simulink model "VehDyn_nstm_model"  (R2023a)
settings: Solver=ode4  StartTime=0.0  StopTime=tend  FixedStep=sample_Ti  RelTol=1e-3
values from neighbouring files (symbols this model uses):
  dpsi_rad_INIT = data.dpsi_radps(1)    [load_nstm_withSimData.m]
  omega_rad_INIT = data.vx_mps(1)/tireFL__MFSIMPLE__r_tire_m    [load_nstm_withSimData.m]
  sample_Ti = 1.e-3    (= 0.001)    [load_nstm_withSimData.m]
  tireFL__MFSIMPLE__r_tire_m = 0.3118    [VehParams.m]
  tireRL__MFSIMPLE__r_tire_m = 0.3118    [VehParams.m]
  VEH__Brakes__d_BrakeActuatorBoreFrRe_m__1 = 0.0798    [VehParams.m]
  VEH__Brakes__d_BrakeActuatorBoreFrRe_m__2 = 0.0798    [VehParams.m]
  VEH__Brakes__mue_BrakePadsFrRe_kinetic__1 = 0.4    [VehParams.m]
  VEH__Brakes__mue_BrakePadsFrRe_kinetic__2 = 0.4    [VehParams.m]
  VEH__Brakes__n_BrakePadsNumberFrRe__1 = 1    [VehParams.m]
  VEH__Brakes__n_BrakePadsNumberFrRe__2 = 1    [VehParams.m]
  VEH__Brakes__r_BrakePadsMeanLeverFrRe_m__1 = 0.134    [VehParams.m]
  VEH__Brakes__r_BrakePadsMeanLeverFrRe_m__2 = 0.134    [VehParams.m]
  VEH__STMspecific__switchModelVel_mps = 3    [VehParams.m]
  vx_INIT = data.vx_mps(1)    [load_nstm_withSimData.m]
  vy_INIT = data.vy_mps(1)    [load_nstm_withSimData.m]
  x0_positionstates = [0 0 0]    [VehParams.m]
  x0_stm_vehiclestates = [0; 0; 0; 0; 0; 0; 0; 0]    [VehParams.m]
settings Model: Creator=ADMIN  LastModifiedBy=ADMIN

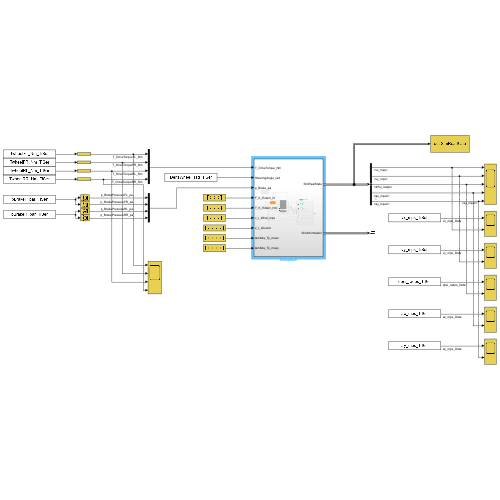
[thumbnail: Simulink's stored preview of the top-level diagram]
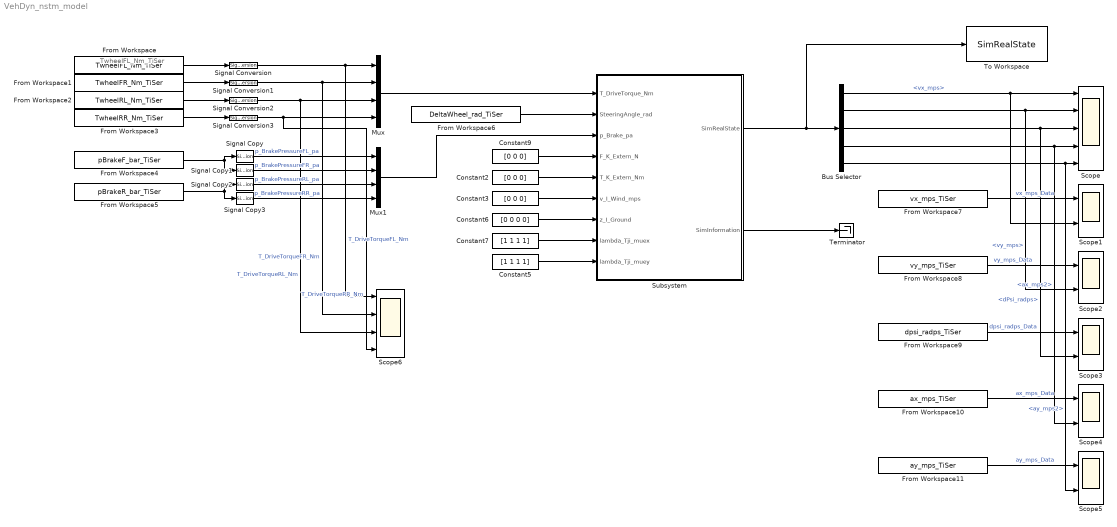
== system VehDyn_nstm_model ==
  note: TwheelFL_Nm_TiSer
  Bus Selector : BusSelector  OutputSignals=vx_mps,vy_mps,dPsi_radps,ax_mps2,ay_mps2
  Constant2 : Constant  Value=[0 0 0]
  Constant3 : Constant  Value=[0 0 0]
  Constant5 : Constant  Value=[1 1 1 1]
  Constant6 : Constant  Value=[0 0 0 0]
  Constant7 : Constant  Value=[1 1 1 1]
  Constant9 : Constant  Value=[0 0 0]
  From Workspace : FromWorkspace  VariableName=TwheelFL_Nm_TiSer  SampleTime=sample_Ti
  From Workspace1 : FromWorkspace  VariableName=TwheelFR_Nm_TiSer  SampleTime=sample_Ti
  From Workspace10 : FromWorkspace  VariableName=ax_mps_TiSer  SampleTime=sample_Ti
  From Workspace11 : FromWorkspace  VariableName=ay_mps_TiSer  SampleTime=sample_Ti
  From Workspace2 : FromWorkspace  VariableName=TwheelRL_Nm_TiSer  SampleTime=sample_Ti
  From Workspace3 : FromWorkspace  VariableName=TwheelRR_Nm_TiSer  SampleTime=sample_Ti
  From Workspace4 : FromWorkspace  VariableName=pBrakeF_bar_TiSer  SampleTime=sample_Ti
  From Workspace5 : FromWorkspace  VariableName=pBrakeR_bar_TiSer  SampleTime=sample_Ti
  From Workspace6 : FromWorkspace  VariableName=DeltaWheel_rad_TiSer  SampleTime=sample_Ti
  From Workspace7 : FromWorkspace  VariableName=vx_mps_TiSer  SampleTime=sample_Ti
  From Workspace8 : FromWorkspace  VariableName=vy_mps_TiSer  SampleTime=sample_Ti
  From Workspace9 : FromWorkspace  VariableName=dpsi_radps_TiSer  SampleTime=sample_Ti
  Mux : Mux
  Mux1 : Mux
  Scope : Scope  NumInputPorts=5
  Scope{1..5} (5 alike) : Scope  NumInputPorts=2
  Scope6 : Scope  NumInputPorts=4
  Signal Conversion{,1..3} (4 alike) : SignalConversion  OverrideOpt=off
  Signal Copy{,1..3} (4 alike) : SignalConversion  OverrideOpt=off
  Subsystem : Subsystem
  Terminator : Terminator
  To Workspace : ToWorkspace  VariableName=SimRealState  SaveFormat=Timeseries  SampleTime=sample_Ti
  wires:
  Signal Copy2/1 -> Mux1/3  "p_BrakePressureRL_pa"
  From Workspace/1 -> Signal Conversion/1
  Mux1/1 -> Subsystem/3(p_Brake_pa)
  From Workspace1/1 -> Signal Conversion1/1
  Signal Conversion/1 -> Scope6/1, Mux/1  "T_DriveTorqueFL_Nm"
  Subsystem/2(SimInformation) -> Terminator/1
  Signal Copy1/1 -> Mux1/2  "p_BrakePressureFR_pa"
  From Workspace3/1 -> Signal Conversion3/1
  From Workspace4/1 -> Signal Copy1/1, Signal Copy/1
  Signal Copy/1 -> Mux1/1  "p_BrakePressureFL_pa"
  From Workspace5/1 -> Signal Copy2/1, Signal Copy3/1
  Bus Selector/1 -> Scope1/2, Scope/1  "<vx_mps>"
  From Workspace2/1 -> Signal Conversion2/1
  Constant2/1 -> Subsystem/5(T_K_Extern_Nm)
  Constant5/1 -> Subsystem/9(lambda_Tji_muey)
  Constant9/1 -> Subsystem/4(F_K_Extern_N)
  Subsystem/1(SimRealState) -> To Workspace/1, Bus Selector/1
  Signal Copy3/1 -> Mux1/4  "p_BrakePressureRR_pa"
  Constant6/1 -> Subsystem/7(z_I_Ground)
  Constant3/1 -> Subsystem/6(v_I_Wind_mps)
  From Workspace6/1 -> Subsystem/2(SteeringAngle_rad)
  Signal Conversion3/1 -> Scope6/4, Mux/4  "T_DriveTorqueRR_Nm"
  Mux/1 -> Subsystem/1(T_DriveTorque_Nm)
  Signal Conversion2/1 -> Scope6/3, Mux/3  "T_DriveTorqueRL_Nm"
  Constant7/1 -> Subsystem/8(lambda_Tji_muex)
  Signal Conversion1/1 -> Scope6/2, Mux/2  "T_DriveTorqueFR_Nm"
  From Workspace7/1 -> Scope1/1  "vx_mps_Data"
  From Workspace8/1 -> Scope2/1  "vy_mps_Data"
  Bus Selector/2 -> Scope2/2, Scope/2  "<vy_mps>"
  From Workspace9/1 -> Scope3/1  "dpsi_radps_Data"
  Bus Selector/3 -> Scope3/2, Scope/3  "<dPsi_radps>"
  Bus Selector/4 -> Scope4/2, Scope/4  "<ax_mps2>"
  From Workspace10/1 -> Scope4/1  "ax_mps_Data"
  From Workspace11/1 -> Scope5/1  "ay_mps_Data"
  Bus Selector/5 -> Scope5/2, Scope/5  "<ay_mps2>"

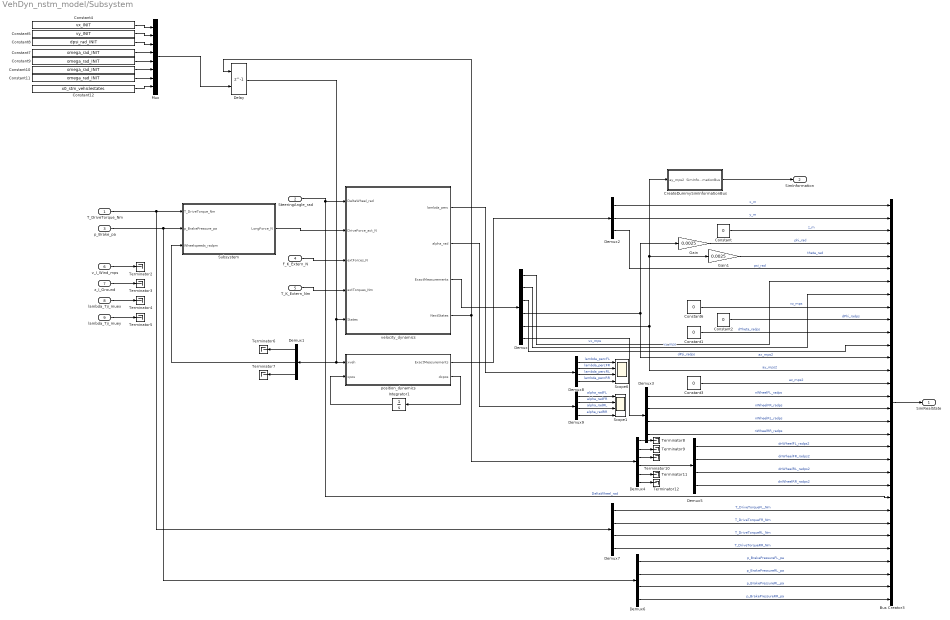
== system VehDyn_nstm_model/Subsystem ==
  T_DriveTorque_Nm : Inport
  SteeringAngle_rad : Inport  Port=2
  p_Brake_pa : Inport  Port=3
  F_K_Extern_N : Inport  Port=4  PortDimensions=3
  T_K_Extern_Nm : Inport  Port=5  PortDimensions=3
  v_I_Wind_mps : Inport  Port=6  PortDimensions=3
  z_I_Ground : Inport  Port=7  PortDimensions=4
  lambda_Tji_muex : Inport  Port=8  PortDimensions=4
  lambda_Tji_muey : Inport  Port=9  PortDimensions=4
  Bus Creator3 : BusCreator  Inputs=32  OutDataTypeStr=Bus: SimRealState
      settings: InheritFromInputs=off
  Constant{,1..3,6} (5 alike) : Constant  Value=0
  Constant{7,9..11} (4 alike) : Constant  Value=omega_rad_INIT
  Constant12 : Constant  Value=x0_stm_vehiclestates
  Constant4 : Constant  Value=vx_INIT
  Constant5 : Constant  Value=vy_INIT
  Constant8 : Constant  Value=dpsi_rad_INIT
  CreateDummySimInformationBus : Subsystem
  Delay : Delay  DelayLength=1  InitialConditionSource=Input port  InitialCondition=0
      settings: InputPortMap=u0,p4
  Demux : Demux  Outputs=[1 1 1 1 1 4]
  Demux1 : Demux  Outputs=[3 4 8]
  Demux2 : Demux  Outputs=3
  Demux{3,5..9} (6 alike) : Demux
  Demux4 : Demux  Outputs=[1 1 1 4 4 4]
  Gain : Gain  Gain=0.0025
  Gain1 : Gain  Gain=0.0025
  Integrator1 : Integrator  InitialCondition=x0_positionstates
  Mux : Mux  Inputs=8
  Scope1 : Scope  NumInputPorts=4
  Scope6 : Scope  NumInputPorts=4
  Subsystem : Subsystem
  Terminator{2..12} (11 alike) : Terminator
  position_dynamics : MATLAB Function  TreatAsAtomicUnit=on
  velocity_dynamics : MATLAB Function  TreatAsAtomicUnit=on
  SimRealState : Outport  OutDataTypeStr=Bus: SimRealState  SampleTime=sample_Ti  VectorParamsAs1DForOutWhenUnconnected=off
  SimInformation : Outport  Port=2  OutDataTypeStr=Bus: SimInformation  VectorParamsAs1DForOutWhenUnconnected=off
  wires:
  Demux2/1 -> Bus Creator3/1  "x_m"
  Demux4/2 -> Terminator9/1
  Constant12/1 -> Mux/8
  Demux/4 -> Gain/1, Bus Creator3/13  "ax_mps2"
  Subsystem/1(LongForce_N) -> velocity_dynamics/2(DriveForce_act_N)
  Bus Creator3/1 -> SimRealState/1
  F_K_Extern_N/1 -> velocity_dynamics/3(extForces_N)
  Constant1/1 -> Bus Creator3/11  "dTheta_radps"
  Demux7/1 -> Bus Creator3/25  "T_DriveTorqueFL_Nm"
  Constant10/1 -> Mux/6
  Constant6/1 -> Bus Creator3/9  "vz_mps"
  Constant8/1 -> Mux/3
  z_I_Ground/1 -> Terminator3/1
  Demux7/4 -> Bus Creator3/28  "T_DriveTorqueRR_Nm"
  Demux7/2 -> Bus Creator3/26  "T_DriveTorqueFR_Nm"
  position_dynamics/1(ExactMeasurements) -> Demux2/1
  Constant4/1 -> Mux/1
  Constant9/1 -> Mux/5
  Demux4/4 -> Demux5/1
  Demux/3 -> Bus Creator3/12  "dPsi_radps"
  Demux6/3 -> Bus Creator3/31  "p_BrakePressureRL_pa"
  CreateDummySimInformationBus/1(SimInformationBus) -> SimInformation/1
  Gain1/1 -> Bus Creator3/5  "theta_rad"
  Constant5/1 -> Mux/2
  Mux/1 -> Delay/2
  p_Brake_pa/1 -> Subsystem/2(p_BrakePressure_pa), Demux6/1
  Demux2/2 -> Bus Creator3/2  "y_m"
  velocity_dynamics/3(ExactMeasurements) -> Demux/1
  Demux5/4 -> Bus Creator3/23  "dnWheelRR_radps2"
  lambda_Tji_muey/1 -> Terminator5/1
  velocity_dynamics/4(NextStates) -> Delay/1, Demux4/1
  Demux1/1 -> Terminator6/1
  Demux4/6 -> Terminator12/1
  Demux4/5 -> Terminator11/1
  Demux4/1 -> Terminator8/1
  lambda_Tji_muex/1 -> Terminator4/1
  Demux3/4 -> Bus Creator3/19  "nWheelRR_radps"
  Demux6/1 -> Bus Creator3/29  "p_BrakePressureFL_pa"
  Demux1/2 -> Subsystem/3(Wheelspeeds_radpm)
  Demux2/3 -> Bus Creator3/6  "psi_rad"
  Demux6/4 -> Bus Creator3/32  "p_BrakePressureRR_pa"
  Constant3/1 -> Bus Creator3/15  "az_mps2"
  Demux6/2 -> Bus Creator3/30  "p_BrakePressureRL_pa"
  Demux5/1 -> Bus Creator3/20  "dnWheelFL_radps2"
  Demux5/2 -> Bus Creator3/21  "dnWheelFR_radps2"
  Demux/1 -> Bus Creator3/7  "vx_mps"
  SteeringAngle_rad/1 -> Bus Creator3/24, velocity_dynamics/1(DeltaWheel_rad)  "DeltaWheel_rad"
  Demux3/2 -> Bus Creator3/17  "nWheelFR_radps"
  Gain/1 -> Bus Creator3/4  "phi_rad"
  Demux3/3 -> Bus Creator3/18  "nWheelRL_radps"
  T_K_Extern_Nm/1 -> velocity_dynamics/4(extTorques_Nm)
  Demux3/1 -> Bus Creator3/16  "nWheelFL_radps"
  Constant/1 -> Bus Creator3/3  "z_m"
  Constant11/1 -> Mux/7
  v_I_Wind_mps/1 -> Terminator2/1
  T_DriveTorque_Nm/1 -> Demux7/1, Subsystem/1(T_DriveTorque_Nm)
  Demux7/3 -> Bus Creator3/27  "T_DriveTorqueRL_Nm"
  Demux/5 -> CreateDummySimInformationBus/1(ay_mps2), Gain1/1, Bus Creator3/14  "ay_mps2"
  Demux5/3 -> Bus Creator3/22  "dnWheelRL_radps2"
  position_dynamics/2(dxpos) -> Integrator1/1
  Integrator1/1 -> position_dynamics/2(xpos)
  Demux1/3 -> Terminator7/1
  Delay/1 -> Demux1/1, position_dynamics/1(xveh), velocity_dynamics/5(States)
  Constant2/1 -> Bus Creator3/10  "dPhi_radps"
  Demux/6 -> Demux3/1
  Constant7/1 -> Mux/4
  Demux4/3 -> Terminator10/1
  Demux/2 -> Bus Creator3/8  "vy_mps"
  velocity_dynamics/1(lambda_perc) -> Demux8/1
  Demux8/1 -> Scope6/1  "lambda_percFL"
  Demux8/2 -> Scope6/2  "lambda_percFR"
  Demux8/3 -> Scope6/3  "lambda_percRL"
  Demux8/4 -> Scope6/4  "lambda_percRR"
  Demux9/3 -> Scope1/3  "alpha_radRL"
  Demux9/2 -> Scope1/2  "alpha_radFR"
  Demux9/4 -> Scope1/4  "alpha_radRR"
  Demux9/1 -> Scope1/1  "alpha_radFL"
  velocity_dynamics/2(alpha_rad) -> Demux9/1

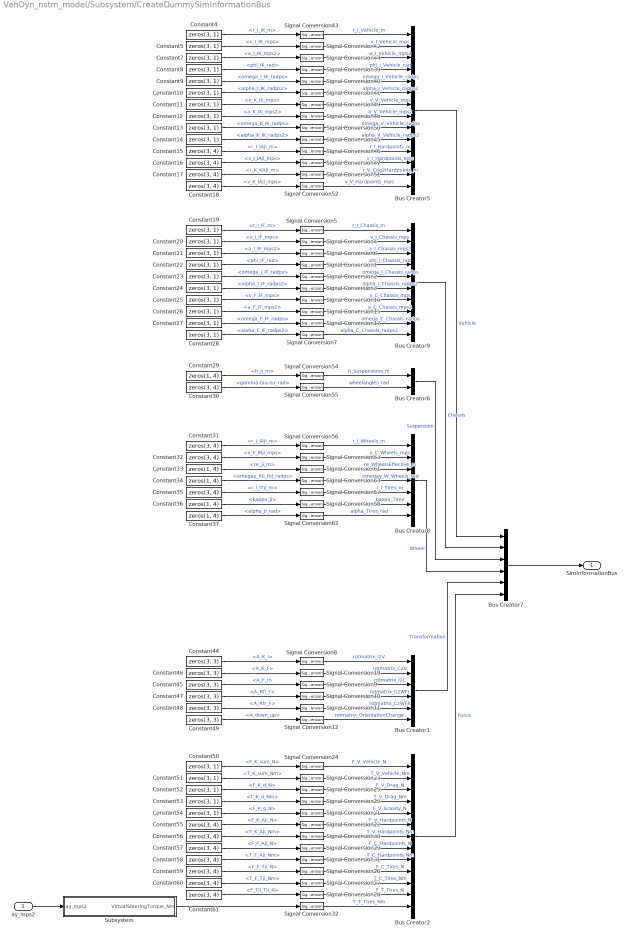
== system VehDyn_nstm_model/Subsystem/CreateDummySimInformationBus ==
  ay_mps2 : Inport
  Bus Creator1 : BusCreator  Inputs=6  OutDataTypeStr=Bus: Transformation
      settings: InheritFromInputs=off
  Bus Creator2 : BusCreator  Inputs=13  OutDataTypeStr=Bus: Force
      settings: InheritFromInputs=off
  Bus Creator5 : BusCreator  Inputs=14  OutDataTypeStr=Bus: Vehicle
      settings: InheritFromInputs=off
  Bus Creator6 : BusCreator  Inputs=2  OutDataTypeStr=Bus: Suspension
      settings: InheritFromInputs=off
  Bus Creator7 : BusCreator  Inputs=6  OutDataTypeStr=Bus: SimInformation
      settings: InheritFromInputs=off
  Bus Creator8 : BusCreator  Inputs=7  OutDataTypeStr=Bus: Wheel
      settings: InheritFromInputs=off
  Bus Creator9 : BusCreator  Inputs=10  OutDataTypeStr=Bus: Chassis
      settings: InheritFromInputs=off
  Constant{4..5,7..14,19..28,50..54} (25 alike) : Constant  Value=zeros(3, 1)
  Constant{15..18,30..32,35,55..61} (15 alike) : Constant  Value=zeros(3, 4)
  Constant{29,33..34,36..37} (5 alike) : Constant  Value=zeros(1, 4)
  Constant{44..49} (6 alike) : Constant  Value=zeros(3, 3)
  Signal Conversion{1..12,15..17,19..32,39..58,61..63} (52 alike) : SignalConversion  OverrideOpt=off
  Subsystem : Subsystem
  SimInformationBus : Outport  VectorParamsAs1DForOutWhenUnconnected=off
  wires:
  Signal Conversion46/1 -> Bus Creator5/11  "r_I_Hardpoints_m"
  Signal Conversion26/1 -> Bus Creator2/10  "F_C_Tires_N"
  Signal Conversion45/1 -> Bus Creator5/10  "alpha_V_Vehicle_radps2"
  Constant33/1 -> Signal Conversion61/1  "<re_ji_m>"
  Signal Conversion15/1 -> Bus Creator9/8  "a_C_Chassis_mps2"
  Signal Conversion58/1 -> Bus Creator8/6  "kappa_Tires"
  Constant60/1 -> Signal Conversion27/1  "<T_F_Tji_Nm>"
  Signal Conversion5/1 -> Bus Creator9/1  "r_I_Chassis_m"
  Signal Conversion17/1 -> Bus Creator9/9  "omega_C_Chassis_radps"
  Signal Conversion8/1 -> Bus Creator1/1  "rotmatrix_I2V"
  Constant13/1 -> Signal Conversion50/1  "<omega_K_IK_radps>"
  Constant24/1 -> Signal Conversion3/1  "<alpha_I_IF_radps2>"
  Signal Conversion16/1 -> Bus Creator9/7  "v_C_Chassis_mps"
  Signal Conversion23/1 -> Bus Creator2/2  "T_V_Vehicle_Nm"
  Signal Conversion3/1 -> Bus Creator9/6  "alpha_I_Chassis_radps2"
  Bus Creator5/1 -> Bus Creator7/1  "Vehicle"
  Signal Conversion32/1 -> Bus Creator2/13  "T_T_Tires_Nm"
  Signal Conversion39/1 -> Bus Creator5/4  "phi_I_Vehicle_rad"
  Signal Conversion29/1 -> Bus Creator2/8  "F_C_Hardpoints_N"
  Constant25/1 -> Signal Conversion16/1  "<v_F_IF_mps>"
  Signal Conversion43/1 -> Bus Creator5/1  "r_I_Vehicle_m"
  Constant47/1 -> Signal Conversion10/1  "<A_Rfl_F>"
  Constant9/1 -> Signal Conversion40/1  "<omega_I_IK_radps>"
  Constant26/1 -> Signal Conversion15/1  "<a_F_IF_mps2>"
  Constant27/1 -> Signal Conversion17/1  "<omega_F_IF_radps>"
  Signal Conversion10/1 -> Bus Creator1/4  "rotmatrix_C2WFL"
  Signal Conversion19/1 -> Bus Creator1/2  "rotmatrix_C2V"
  Constant7/1 -> Signal Conversion44/1  "<a_I_IK_mps2>"
  Bus Creator8/1 -> Bus Creator7/4  "Wheel"
  Signal Conversion9/1 -> Bus Creator1/3  "rotmatrix_I2C"
  Signal Conversion31/1 -> Bus Creator2/9  "T_C_Hardpoints_Nm"
  Signal Conversion62/1 -> Bus Creator8/7  "alpha_Tires_rad"
  Signal Conversion30/1 -> Bus Creator2/7  "T_V_Hardpoints_Nm"
  Signal Conversion48/1 -> Bus Creator5/8  "a_V_Vehicle_mps2"
  Signal Conversion54/1 -> Bus Creator6/1  "h_Suspensions_m"
  Signal Conversion56/1 -> Bus Creator8/1  "r_I_Wheels_m"
  Signal Conversion7/1 -> Bus Creator9/10  "alpha_C_Chassis_radps2"
  Signal Conversion12/1 -> Bus Creator1/6  "rotmatrix_OrientationChange"
  Signal Conversion21/1 -> Bus Creator2/5  "F_V_Gravity_N"
  Signal Conversion53/1 -> Bus Creator8/2  "v_C_Wheels_mps"
  Signal Conversion22/1 -> Bus Creator2/6  "F_V_Hardpoints_N"
  Signal Conversion27/1 -> Bus Creator2/11  "T_C_Tires_Nm"
  Signal Conversion51/1 -> Bus Creator5/13  "r_V_Cog2Hardpoints_m"
  Constant28/1 -> Signal Conversion7/1  "<alpha_F_IF_radps2>"
  Signal Conversion55/1 -> Bus Creator6/2  "wheelangles_rad"
  Signal Conversion57/1 -> Bus Creator8/5  "r_I_Tires_m"
  Signal Conversion4/1 -> Bus Creator9/2  "v_I_Chassis_mps"
  Bus Creator2/1 -> Bus Creator7/6  "Force"
  Signal Conversion20/1 -> Bus Creator2/4  "T_V_Drag_Nm"
  Signal Conversion40/1 -> Bus Creator5/5  "omega_I_Vehicle_radps"
  Bus Creator1/1 -> Bus Creator7/5  "Transformation"
  Signal Conversion41/1 -> Bus Creator5/6  "alpha_I_Vehicle_radps2"
  Bus Creator9/1 -> Bus Creator7/2  "Chassis"
  Signal Conversion6/1 -> Bus Creator9/3  "a_I_Chassis_mps2"
  Bus Creator6/1 -> Bus Creator7/3  "Suspension"
  Signal Conversion61/1 -> Bus Creator8/3  "re_WheelsEffective_m"
  Signal Conversion44/1 -> Bus Creator5/3  "a_I_Vehicle_mps2"
  Signal Conversion42/1 -> Bus Creator5/2  "v_I_Vehicle_mps"
  Signal Conversion63/1 -> Bus Creator8/4  "omegay_W_Wheels_rad"
  Constant31/1 -> Signal Conversion56/1  "<r_I_IRji_m>"
  Signal Conversion49/1 -> Bus Creator5/7  "v_V_Vehicle_mps"
  Signal Conversion28/1 -> Bus Creator2/12  "F_T_Tires_N"
  Signal Conversion11/1 -> Bus Creator1/5  "rotmatrix_C2WFR"
  Signal Conversion50/1 -> Bus Creator5/9  "omega_V_Vehicle_radps"
  Signal Conversion24/1 -> Bus Creator2/1  "F_V_Vehicle_N"
  Constant19/1 -> Signal Conversion5/1  "<r_I_IF_m>"
  Constant22/1 -> Signal Conversion1/1  "<phi_IF_rad>"
  Constant11/1 -> Signal Conversion49/1  "<v_K_IK_mps>"
  Constant58/1 -> Signal Conversion31/1  "<T_F_Aji_Nm>"
  Constant20/1 -> Signal Conversion4/1  "<v_I_IF_mps>"
  Constant44/1 -> Signal Conversion8/1  "<A_K_I>"
  Constant36/1 -> Signal Conversion58/1  "<kappa_ji>"
  Constant32/1 -> Signal Conversion53/1  "<v_F_IRji_mps>"
  Constant8/1 -> Signal Conversion39/1  "<phi_IK_rad>"
  Signal Conversion2/1 -> Bus Creator9/5  "omega_I_Chassis_radps"
  Constant5/1 -> Signal Conversion42/1  "<v_I_IK_mps>"
  Constant10/1 -> Signal Conversion41/1  "<alpha_I_IK_radps2>"
  Constant4/1 -> Signal Conversion43/1  "<r_I_IK_m>"
  Constant29/1 -> Signal Conversion54/1  "<h_ji_m>"
  Subsystem/1(VirtualSteeringTorque_Nm) -> Signal Conversion32/1
  Constant35/1 -> Signal Conversion57/1  "<r_I_ITji_m>"
  Signal Conversion47/1 -> Bus Creator5/12  "v_I_Hardpoints_mps"
  Constant57/1 -> Signal Conversion29/1  "<F_F_Aji_N>"
  Constant48/1 -> Signal Conversion11/1  "<A_Rfr_F>"
  Constant50/1 -> Signal Conversion24/1  "<F_K_sum_N>"
  Constant53/1 -> Signal Conversion20/1  "<T_K_d_Nm>"
  Constant49/1 -> Signal Conversion12/1  "<A_down_up>"
  Constant51/1 -> Signal Conversion23/1  "<T_K_sum_Nm>"
  Constant12/1 -> Signal Conversion48/1  "<a_K_IK_mps2>"
  Constant15/1 -> Signal Conversion46/1  "<r_I_IAji_m>"
  Constant54/1 -> Signal Conversion21/1  "<F_K_g_N>"
  Constant17/1 -> Signal Conversion51/1  "<r_K_KAji_m>"
  Constant55/1 -> Signal Conversion22/1  "<F_K_Aji_N>"
  Constant21/1 -> Signal Conversion6/1  "<a_I_IF_mps2>"
  Constant52/1 -> Signal Conversion25/1  "<F_K_d_N>"
  Constant30/1 -> Signal Conversion55/1  "<gamma-tau-nu_rad>"
  Constant14/1 -> Signal Conversion45/1  "<alpha_K_IK_radps2>"
  Constant18/1 -> Signal Conversion52/1  "<v_K_IAji_mps>"
  Constant59/1 -> Signal Conversion26/1  "<F_F_Tji_N>"
  Constant61/1 -> Signal Conversion28/1  "<F_Tji_Tji_N>"
  Constant56/1 -> Signal Conversion30/1  "<T_K_Aji_Nm>"
  Constant37/1 -> Signal Conversion62/1  "<alpha_ji_rad>"
  Constant34/1 -> Signal Conversion63/1  "<omegay_Rji_Rji_radps>"
  Constant45/1 -> Signal Conversion9/1  "<A_F_I>"
  Signal Conversion1/1 -> Bus Creator9/4  "phi_I_Chassis_rad"
  Signal Conversion52/1 -> Bus Creator5/14  "v_V_Hardpoints_mps"
  Constant46/1 -> Signal Conversion19/1  "<A_K_F>"
  Constant23/1 -> Signal Conversion2/1  "<omega_I_IF_radps>"
  Constant16/1 -> Signal Conversion47/1  "<v_I_IAji_mps>"
  Signal Conversion25/1 -> Bus Creator2/3  "F_V_Drag_N"
  Bus Creator7/1 -> SimInformationBus/1
  ay_mps2/1 -> Subsystem/1(ay_mps2)

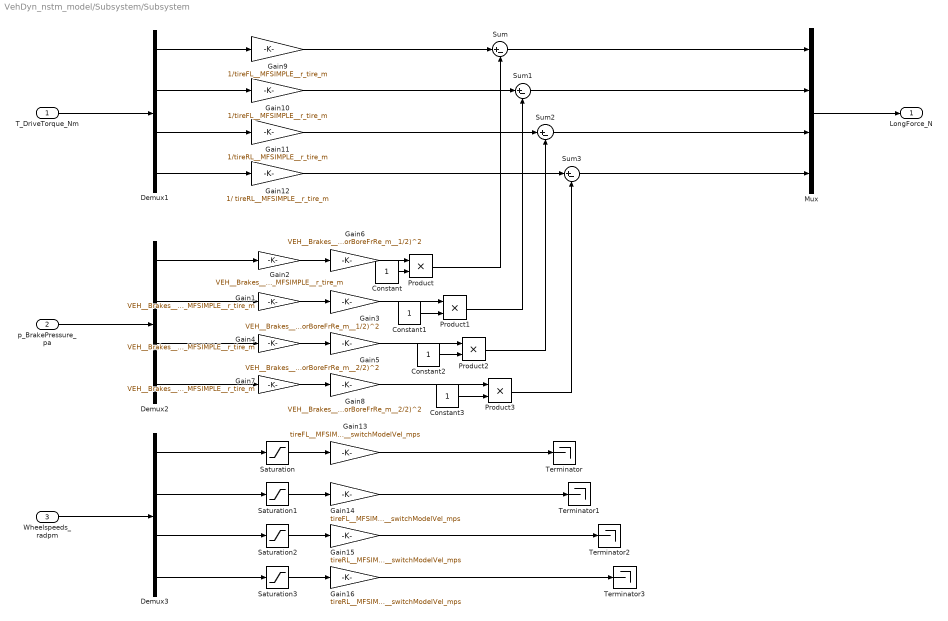
== system VehDyn_nstm_model/Subsystem/Subsystem ==
  T_DriveTorque_Nm : Inport
  p_BrakePressure_pa : Inport  Port=2
  Wheelspeeds_radpm : Inport  Port=3
  Constant{,1..3} (4 alike) : Constant
  Demux1 : Demux
  Demux2 : Demux
  Demux3 : Demux
  Gain1 : Gain  Gain=VEH__Brakes__r_BrakePadsMeanLeverFrRe_m__1 / tireFL__MFSIMPLE__r_tire_m
  Gain10 : Gain  Gain=1/tireFL__MFSIMPLE__r_tire_m
  Gain11 : Gain  Gain=1/tireRL__MFSIMPLE__r_tire_m
  Gain12 : Gain  Gain=1/ tireRL__MFSIMPLE__r_tire_m
  Gain13 : Gain  Gain=tireFL__MFSIMPLE__r_tire_m / VEH__STMspecific__switchModelVel_mps
  Gain14 : Gain  Gain=tireFL__MFSIMPLE__r_tire_m / VEH__STMspecific__switchModelVel_mps
  Gain15 : Gain  Gain=tireRL__MFSIMPLE__r_tire_m / VEH__STMspecific__switchModelVel_mps
  Gain16 : Gain  Gain=tireRL__MFSIMPLE__r_tire_m / VEH__STMspecific__switchModelVel_mps
  Gain2 : Gain  Gain=VEH__Brakes__r_BrakePadsMeanLeverFrRe_m__1 / tireFL__MFSIMPLE__r_tire_m
  Gain3 : Gain  Gain=VEH__Brakes__n_BrakePadsNumberFrRe__1 * VEH__Brakes__mue_BrakePadsFrRe_kinetic__1 * pi * (VEH__Brakes__d_BrakeActuatorBoreFrRe_m__1/2)^2
  Gain4 : Gain  Gain=VEH__Brakes__r_BrakePadsMeanLeverFrRe_m__2 / tireRL__MFSIMPLE__r_tire_m
  Gain5 : Gain  Gain=VEH__Brakes__n_BrakePadsNumberFrRe__2 * VEH__Brakes__mue_BrakePadsFrRe_kinetic__2 * pi * (VEH__Brakes__d_BrakeActuatorBoreFrRe_m__2/2)^2
  Gain6 : Gain  Gain=VEH__Brakes__n_BrakePadsNumberFrRe__1 * VEH__Brakes__mue_BrakePadsFrRe_kinetic__1 * pi * (VEH__Brakes__d_BrakeActuatorBoreFrRe_m__1/2)^2
  Gain7 : Gain  Gain=VEH__Brakes__r_BrakePadsMeanLeverFrRe_m__2 / tireRL__MFSIMPLE__r_tire_m
  Gain8 : Gain  Gain=VEH__Brakes__n_BrakePadsNumberFrRe__2 * VEH__Brakes__mue_BrakePadsFrRe_kinetic__2 * pi * (VEH__Brakes__d_BrakeActuatorBoreFrRe_m__2/2)^2
  Gain9 : Gain  Gain=1/tireFL__MFSIMPLE__r_tire_m
  Mux : Mux
  Product{,1..3} (4 alike) : Product
  Saturation : Saturate  UpperLimit=VEH__STMspecific__switchModelVel_mps / tireFL__MFSIMPLE__r_tire_m  LowerLimit=0
  Saturation1 : Saturate  UpperLimit=VEH__STMspecific__switchModelVel_mps / tireFL__MFSIMPLE__r_tire_m  LowerLimit=0
  Saturation2 : Saturate  UpperLimit=VEH__STMspecific__switchModelVel_mps / tireRL__MFSIMPLE__r_tire_m  LowerLimit=0
  Saturation3 : Saturate  UpperLimit=VEH__STMspecific__switchModelVel_mps / tireRL__MFSIMPLE__r_tire_m  LowerLimit=0
  Sum{,1..3} (4 alike) : Sum  Inputs=|+-
  Terminator{,1..3} (4 alike) : Terminator
  LongForce_N : Outport  VectorParamsAs1DForOutWhenUnconnected=off
  wires:
  Demux1/4 -> Gain12/1
  Gain9/1 -> Sum/1
  Product2/1 -> Sum2/2
  Demux2/4 -> Gain7/1
  Mux/1 -> LongForce_N/1
  T_DriveTorque_Nm/1 -> Demux1/1
  Demux1/3 -> Gain11/1
  Demux1/1 -> Gain9/1
  Gain4/1 -> Gain5/1
  Gain2/1 -> Gain6/1
  Sum3/1 -> Mux/4
  Demux2/1 -> Gain2/1
  Product3/1 -> Sum3/2
  Gain11/1 -> Sum2/1
  Gain10/1 -> Sum1/1
  Demux2/2 -> Gain1/1
  Sum1/1 -> Mux/2
  Sum/1 -> Mux/1
  Demux1/2 -> Gain10/1
  Gain1/1 -> Gain3/1
  Gain7/1 -> Gain8/1
  p_BrakePressure_pa/1 -> Demux2/1
  Gain12/1 -> Sum3/1
  Demux2/3 -> Gain4/1
  Sum2/1 -> Mux/3
  Product/1 -> Sum/2
  Product1/1 -> Sum1/2
  Wheelspeeds_radpm/1 -> Demux3/1
  Demux3/1 -> Saturation/1
  Demux3/2 -> Saturation1/1
  Demux3/3 -> Saturation2/1
  Demux3/4 -> Saturation3/1
  Saturation/1 -> Gain13/1
  Saturation1/1 -> Gain14/1
  Saturation2/1 -> Gain15/1
  Saturation3/1 -> Gain16/1
  Gain6/1 -> Product/1
  Gain13/1 -> Terminator/1
  Gain3/1 -> Product1/1
  Gain14/1 -> Terminator1/1
  Gain5/1 -> Product2/1
  Gain15/1 -> Terminator2/1
  Gain8/1 -> Product3/1
  Gain16/1 -> Terminator3/1
  Constant/1 -> Product/2
  Constant1/1 -> Product1/2
  Constant2/1 -> Product2/2
  Constant3/1 -> Product3/2

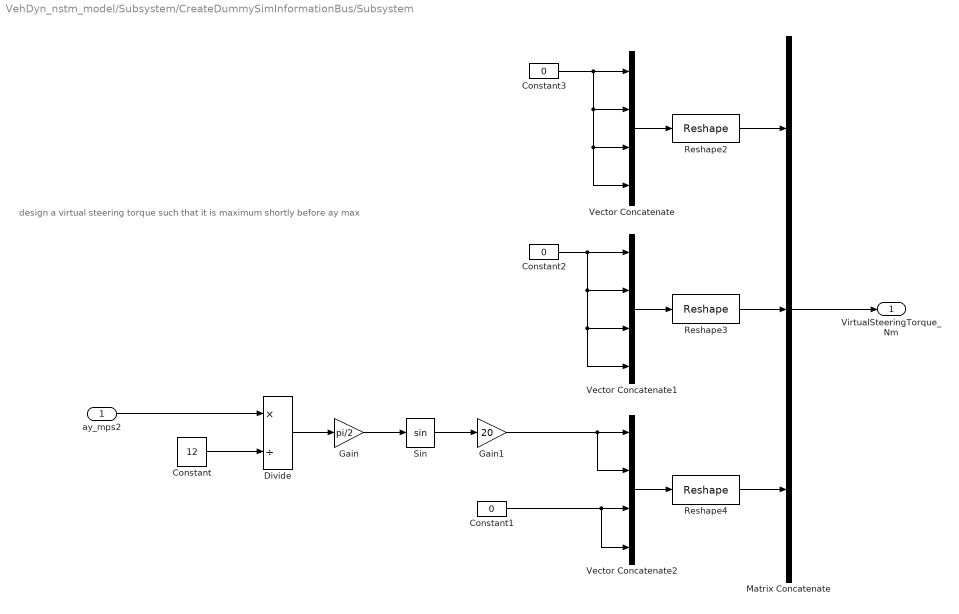
== system VehDyn_nstm_model/Subsystem/CreateDummySimInformationBus/Subsystem ==
  note: design a virtual steering torque such that it is maximum shortly before ay max
  ay_mps2 : Inport
  Constant : Constant  Value=12
  Constant1 : Constant  Value=0
  Constant2 : Constant  Value=0
  Constant3 : Constant  Value=0
  Divide : Product  Inputs=*/
  Gain : Gain  Gain=pi/2
  Gain1 : Gain  Gain=20
  Matrix Concatenate : Concatenate  NumInputs=3  Mode=Multidimensional array
  Reshape2 : Reshape  OutputDimensionality=Row vector (2-D)
  Reshape3 : Reshape  OutputDimensionality=Row vector (2-D)
  Reshape4 : Reshape  OutputDimensionality=Row vector (2-D)
  Sin : Trigonometry
  Vector Concatenate : Concatenate  NumInputs=4
  Vector Concatenate1 : Concatenate  NumInputs=4
  Vector Concatenate2 : Concatenate  NumInputs=4
  VirtualSteeringTorque_Nm : Outport  VectorParamsAs1DForOutWhenUnconnected=off
  wires:
  ay_mps2/1 -> Divide/1
  Constant/1 -> Divide/2
  Divide/1 -> Gain/1
  Gain/1 -> Sin/1
  Sin/1 -> Gain1/1
  Constant3/1 -> Vector Concatenate/4, Vector Concatenate/3, Vector Concatenate/2, Vector Concatenate/1
  Reshape3/1 -> Matrix Concatenate/2
  Reshape4/1 -> Matrix Concatenate/3
  Vector Concatenate1/1 -> Reshape3/1
  Constant1/1 -> Vector Concatenate2/4, Vector Concatenate2/3
  Vector Concatenate2/1 -> Reshape4/1
  Vector Concatenate/1 -> Reshape2/1
  Constant2/1 -> Vector Concatenate1/4, Vector Concatenate1/3, Vector Concatenate1/2, Vector Concatenate1/1
  Gain1/1 -> Vector Concatenate2/2, Vector Concatenate2/1
  Reshape2/1 -> Matrix Concatenate/1
  Matrix Concatenate/1 -> VirtualSteeringTorque_Nm/1

== matlab function VehDyn_nstm_model/Subsystem/velocity_dynamics ==
  data: lambda_perc output; alpha_rad output; ExactMeasurements output; DeltaWheel_rad input; DriveForce_act_N input size=4; extForces_N input; extTorques_Nm input; NextStates output; States input; VEH__VehicleData__w_TrackF_m parameter; VEH__VehicleData__w_TrackR_m parameter; VEH__VehicleData__l_WheelbaseF_m parameter; VEH__VehicleData__l_WheelbaseTotal_m parameter; VEH__VehicleData__m_Vehicle_kg parameter; VEH__VehicleData__I_K_Vehicle_kgm2__33 parameter; VEH__Aerodynamics__A_LongitudinalDrag_m2 parameter; VEH__Aerodynamics__cw_LongitudinalDrag parameter; VEH__STMspecific__cLiftF parameter; VEH__STMspecific__cLiftR parameter; VEH__STMspecific__cRollFriction_Npmps parameter; VEH__STMspecific__MaxRollFriction_N parameter; tireFL__MFSIMPLE__PacLong_B parameter; tireFL__MFSIMPLE__PacLong_C parameter; tireFL__MFSIMPLE__PacLong_D parameter; tireFL__MFSIMPLE__PacLong_E parameter; tireFL__MFSIMPLE__PacLong_Fznom parameter; tireFL__MFSIMPLE__PacLat_B parameter; tireFL__MFSIMPLE__PacLat_C parameter; tireFL__MFSIMPLE__PacLat_D parameter; tireFL__MFSIMPLE__PacLat_E parameter; tireFL__MFSIMPLE__PacLat_Fznom parameter; tireFL__MFSIMPLE__r_tire_m parameter; tireFL__MFSIMPLE__Iyy_Wheel_kgm2 parameter; tireRL__MFSIMPLE__PacLong_B parameter; tireRL__MFSIMPLE__PacLong_C parameter; tireRL__MFSIMPLE__PacLong_D parameter; tireRL__MFSIMPLE__PacLong_E parameter; tireRL__MFSIMPLE__PacLong_Fznom parameter; tireRL__MFSIMPLE__PacLat_B parameter; tireRL__MFSIMPLE__PacLat_C parameter; tireRL__MFSIMPLE__PacLat_D parameter; tireRL__MFSIMPLE__PacLat_E parameter; tireRL__MFSIMPLE__PacLat_Fznom parameter; tireRL__MFSIMPLE__r_tire_m parameter; tireRL__MFSIMPLE__Iyy_Wheel_kgm2 parameter; VEH__STMspecific__PTLimitLowVel_N parameter; VEH__STMspecific__switchModelBlend_mps parameter; VEH__STMspecific__switchModelVel_mps parameter; VEH__STMspecific__T_LatVel_s parameter; VEH__STMspecific__T_Tire_s parameter; VEH__STMspecific__T_YawRate_s parameter; tireFL__MFSIMPLE__PacLat_eps_load parameter; tireFL__MFSIMPLE__PacLong_eps_load parameter; tireRL__MFSIMPLE__PacLat_eps_load parameter; tireRL__MFSIMPLE__PacLong_eps_load parameter; sample_Ti parameter
 function [lambda_perc,alpha_rad, ExactMeasurements, NextStates] = fcn(DeltaWheel_rad, DriveForce_act_N, extForces_N, extTorques_Nm, States, ...
    VEH__VehicleData__w_TrackF_m, VEH__VehicleData__w_TrackR_m, ...
    VEH__VehicleData__l_WheelbaseF_m, VEH__VehicleData__l_WheelbaseTotal_m, ...
    VEH__VehicleData__m_Vehicle_kg, ...
    VEH__VehicleData__I_K_Vehicle_kgm2__33, ...
    VEH__Aerodynamics__A_LongitudinalDrag_m2, VEH__Aerodynamics__cw_LongitudinalDrag, VEH__STMspecific__cLiftF, VEH__STMspecific__cLiftR, ...
    VEH__STMspecific__cRollFriction_Npmps, VEH__STMspecific__MaxRollFriction_N, ...
    tireFL__MFSIMPLE__PacLong_B, tireFL__MFSIMPLE__PacLong_C, tireFL__MFSIMPLE__PacLong_D, tireFL__MFSIMPLE__PacLong_E, tireFL__MFSIMPLE__PacLong_Fznom, tireFL__MFSIMPLE__PacLat_B, tireFL__MFSIMPLE__PacLat_C, tireFL__MFSIMPLE__PacLat_D, tireFL__MFSIMPLE__PacLat_E, tireFL__MFSIMPLE__PacLat_Fznom, tireFL__MFSIMPLE__r_tire_m, tireFL__MFSIMPLE__Iyy_Wheel_kgm2, ...
    tireRL__MFSIMPLE__PacLong_B, tireRL__MFSIMPLE__PacLong_C, tireRL__MFSIMPLE__PacLong_D, tireRL__MFSIMPLE__PacLong_E, tireRL__MFSIMPLE__PacLong_Fznom, tireRL__MFSIMPLE__PacLat_B, tireRL__MFSIMPLE__PacLat_C, tireRL__MFSIMPLE__PacLat_D, tireRL__MFSIMPLE__PacLat_E, tireRL__MFSIMPLE__PacLat_Fznom, tireRL__MFSIMPLE__r_tire_m, tireRL__MFSIMPLE__Iyy_Wheel_kgm2, ...
    VEH__STMspecific__PTLimitLowVel_N, VEH__STMspecific__switchModelBlend_mps, VEH__STMspecific__switchModelVel_mps, ...
    VEH__STMspecific__T_LatVel_s, VEH__STMspecific__T_Tire_s, VEH__STMspecific__T_YawRate_s, ...
    tireFL__MFSIMPLE__PacLat_eps_load, ...
    tireFL__MFSIMPLE__PacLong_eps_load, ...
    tireRL__MFSIMPLE__PacLat_eps_load, ... 
    tireRL__MFSIMPLE__PacLong_eps_load, ...
sample_Ti)


    %% parameter mapping

        veh_param.tw_front_m = VEH__VehicleData__w_TrackF_m; 
        veh_param.tw_rear_m = VEH__VehicleData__w_TrackR_m; 
        veh_param.l_front_m = VEH__VehicleData__l_WheelbaseF_m; 
        veh_param.l_total_m = VEH__VehicleData__l_WheelbaseTotal_m;
        veh_param.m_Vehicle_kg = VEH__VehicleData__m_Vehicle_kg; 
        veh_param.VehicleInertia_kgm2 = VEH__VehicleData__I_K_Vehicle_kgm2__33;

        veh_param.T_LatVel_s = VEH__STMspecific__T_LatVel_s; 
        veh_param.T_YawRate_s = VEH__STMspecific__T_YawRate_s; 
        veh_param.cDrag = VEH__Aerodynamics__cw_LongitudinalDrag; 
        veh_param.Aref_m2 = VEH__Aerodynamics__A_LongitudinalDrag_m2;

        veh_param.cRollFriction_Npmps = VEH__STMspecific__cRollFriction_Npmps;

        veh_param.PacLatF = [tireFL__MFSIMPLE__PacLat_B, tireFL__MFSIMPLE__PacLat_C, tireFL__MFSIMPLE__PacLat_D, tireFL__MFSIMPLE__PacLat_E, tireFL__MFSIMPLE__PacLat_Fznom, tireFL__MFSIMPLE__PacLat_eps_load];
        veh_param.PacLatR = [tireRL__MFSIMPLE__PacLat_B, tireRL__MFSIMPLE__PacLat_C, tireRL__MFSIMPLE__PacLat_D, tireRL__MFSIMPLE__PacLat_E, tireRL__MFSIMPLE__PacLat_Fznom, tireRL__MFSIMPLE__PacLat_eps_load];
        veh_param.PacLongF = [tireFL__MFSIMPLE__PacLong_B, tireFL__MFSIMPLE__PacLong_C, tireFL__MFSIMPLE__PacLong_D, tireFL__MFSIMPLE__PacLong_E, tireFL__MFSIMPLE__PacLong_Fznom, tireFL__MFSIMPLE__PacLong_eps_load];
        veh_param.PacLongR = [tireRL__MFSIMPLE__PacLong_B, tireRL__MFSIMPLE__PacLong_C, tireRL__MFSIMPLE__PacLong_D, tireRL__MFSIMPLE__PacLong_E, tireRL__MFSIMPLE__PacLong_Fznom, tireRL__MFSIMPLE__PacLong_eps_load];
        veh_param.r_tireF_m = tireFL__MFSIMPLE__r_tire_m;
        veh_param.r_tireR_m = tireRL__MFSIMPLE__r_tire_m;
        veh_param.WheelInertiaF_kgm2 = tireFL__MFSIMPLE__Iyy_Wheel_kgm2;
        veh_param.WheelInertiaR_kgm2 = tireRL__MFSIMPLE__Iyy_Wheel_kgm2;

        veh_param.MaxRollFriction_N = VEH__STMspecific__MaxRollFriction_N;
        veh_param.switchModelVel_mps = VEH__STMspecific__switchModelVel_mps; 
        veh_param.switchModelBlend_mps = VEH__STMspecific__switchModelBlend_mps; 
        veh_param.PTLimitLowVel_N = VEH__STMspecific__PTLimitLowVel_N; 
        veh_param.T_Tire_s = VEH__STMspecific__T_Tire_s; 
        veh_param.cLiftF = VEH__STMspecific__cLiftF;
        veh_param.cLiftR = VEH__STMspecific__cLiftR;

    %% function call
    [lambda_perc,alpha_rad, ExactMeasurements, NextStates] = VehicleModel(DeltaWheel_rad, DriveForce_act_N, extForces_N, extTorques_Nm, States, veh_param, sample_Ti);

== matlab function VehDyn_nstm_model/Subsystem/position_dynamics ==
  data: ExactMeasurements output; xveh input; xpos input; dxpos output
function [ExactMeasurements, dxpos] = fcn(xveh, xpos)

[ExactMeasurements, dxpos] = PositionModel(xveh, xpos);
